simulink model "simFWD_1dof"  (R2021b)
settings: Solver=FixedStepAuto  StartTime=0.0  StopTime=simTime  FixedStep=samplingPeriod/500
values from neighbouring files (symbols this model uses):
  drv = driveNo3    [id_1dof_dyn.m]    (also in id_1dof_static.m)
  dwellTimeInit = 0    [id_1dof_dyn.m]
  frictionInit = Transmission.getFrictionCoeff(velocityInit, kinFriction, strbInf, strbVelocity)    [id_1dof_dyn.m]
  loadInertia = mass*pulleyRad^2    (= 3.84e-05)    [id_1dof_dyn.m]    (also in id_1dof_static.m)
  payload = gravity*mass*pulleyRad    (= 0.01883904)    [id_1dof_dyn.m]    (also in id_1dof_static.m)
  velocityInit = mean(expVelocity(1:5))    [id_1dof_dyn.m]
settings Model: Creator=anestis  LastModifiedBy=Anestis Mablekos
settings SolverCC: AlgebraicLoopSolver=TrustRegion  SolverResetMethod=Robust
settings DataIOCC: ReturnWorkspaceOutputs=off
settings DebuggingCC: SFMachineParentedDataDiag=warning  ArithmeticOperatorsInVariantConditions=warning
settings SFSimCC: SimUseLocalCustomCode=off  CustomCodeUndefinedFunction=UseInterfaceOnly
settings RTWCC: RTWUseLocalCustomCode=off
settings CodeAppCC: StateflowObjectComments=on

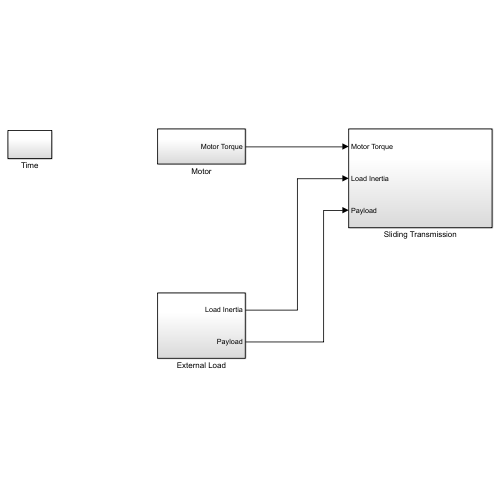
[thumbnail: Simulink's stored preview of the top-level diagram]
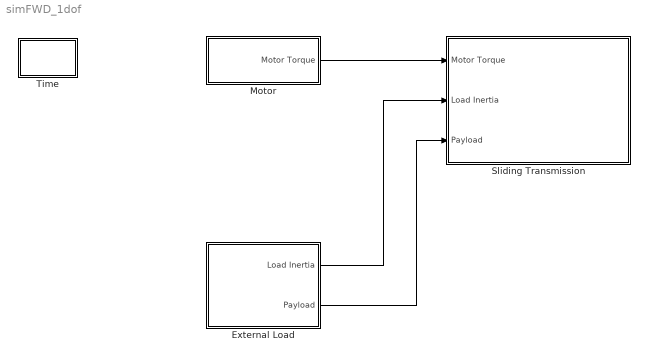
== system simFWD_1dof ==
  External Load : Subsystem
  Motor : Subsystem
  Sliding Transmission : Subsystem
  Time : Subsystem
  wires:
  External Load/1(Load Inertia) -> Sliding Transmission/2(Load Inertia)
  External Load/2(Payload) -> Sliding Transmission/3(Payload)
  Motor/1(Motor Torque) -> Sliding Transmission/1(Motor Torque)

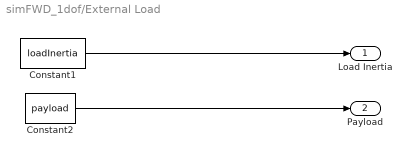
== system simFWD_1dof/External Load ==
  Constant1 : Constant  Value=loadInertia
  Constant2 : Constant  Value=payload
  Load Inertia : Outport
  Payload : Outport  Port=2
  wires:
  Constant1/1 -> Load Inertia/1
  Constant2/1 -> Payload/1

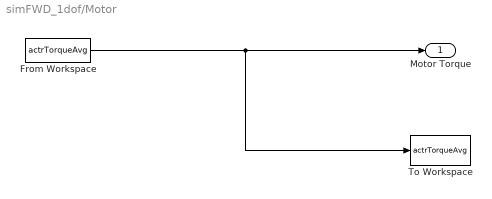
== system simFWD_1dof/Motor ==
  From Workspace : FromWorkspace  VariableName=actrTorqueAvg
  To Workspace : ToWorkspace  VariableName=actrTorqueAvg  SaveFormat=Timeseries  SampleTime=-1
  Motor Torque : Outport
  wires:
  From Workspace/1 -> To Workspace/1, Motor Torque/1

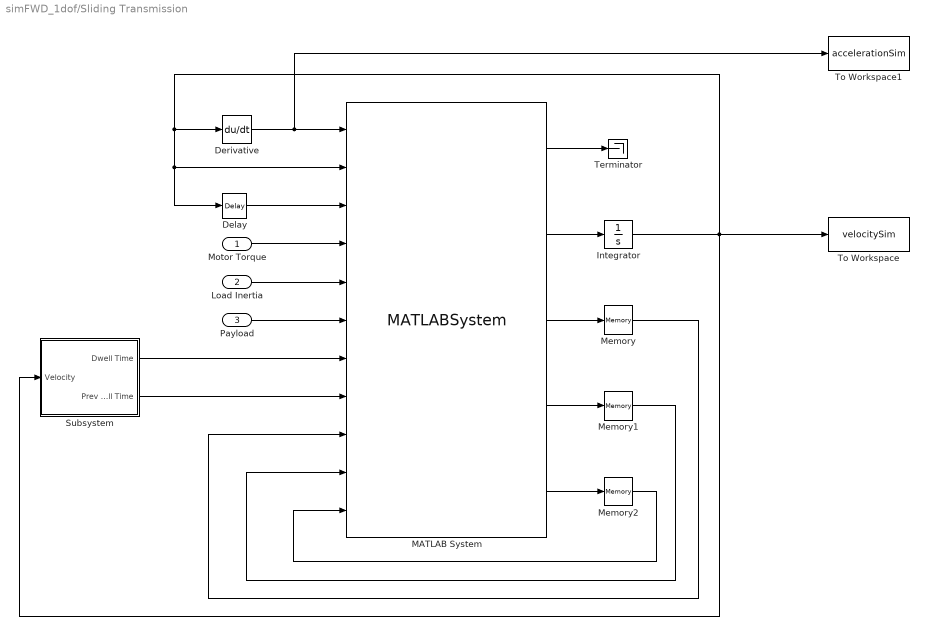
== system simFWD_1dof/Sliding Transmission ==
  Motor Torque : Inport
  Load Inertia : Inport  Port=2
  Payload : Inport  Port=3
  Delay : TransportDelay  DelayTime=drv.friction.memoryCst  InitialOutput=velocityInit
  Derivative : Derivative
  Integrator : Integrator
  MATLAB System : MATLABSystem  System=Transmission  geometry=drv.geometry  preload=drv.preload  friction=drv.friction  inertia=drv.inertia  actuation=drv.actuation  SimulateUsing=Code generation
      mask Type: Transmission
      mask Display:
      | disp('Transmission');
      | port_label('input',1,'acceleration');
      | port_label('input',2,'velocity');
      | port_label('input',3,'velocityD');
      | port_label('input',4,'actrTorque');
      | port_label('input',5,'loadInertia');
      | port_label('input',6,'payload');
      | port_label('input',7,'dwellTime');
      | port_label('input',8,'dwellTimePrev');
      | port_label('input',9,'frictionCoeffPrev');
      | port_label('input',10,'strbFrictionPrev');
      | port_label('input',11,'strbArrivalPrev');
      | port_label('output',1,'torque');
      | port_label('output',2,'acceleration');
      | port_label('output',3,'frictionCoeff');
      | port_label('output',4,'strbFriction');
      | port_label('output',5,'strbArrival');
  Memory : Memory  InitialCondition=frictionInit
  Memory1 : Memory  InitialCondition=drv.friction.strbInf
  Memory2 : Memory  InitialCondition=drv.friction.strbInf
  Subsystem : Subsystem
  Terminator : Terminator
  To Workspace : ToWorkspace  VariableName=velocitySim  SaveFormat=Timeseries  SampleTime=-1
  To Workspace1 : ToWorkspace  VariableName=accelerationSim  SaveFormat=Timeseries  SampleTime=-1
  wires:
  Motor Torque/1 -> MATLAB System/4
  Load Inertia/1 -> MATLAB System/5
  Payload/1 -> MATLAB System/6
  Memory/1 -> MATLAB System/9
  Memory1/1 -> MATLAB System/10
  Delay/1 -> MATLAB System/3
  Memory2/1 -> MATLAB System/11
  Integrator/1 -> Subsystem/1(Velocity), To Workspace/1, Delay/1, MATLAB System/2, Derivative/1
  Derivative/1 -> To Workspace1/1, MATLAB System/1
  MATLAB System/5 -> Memory2/1
  MATLAB System/3 -> Memory/1
  MATLAB System/2 -> Integrator/1
  MATLAB System/1 -> Terminator/1
  MATLAB System/4 -> Memory1/1
  Subsystem/1(Dwell Time) -> MATLAB System/7
  Subsystem/2(Prev Dwell Time) -> MATLAB System/8

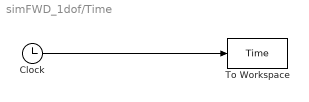
== system simFWD_1dof/Time ==
  Clock : Clock
  To Workspace : ToWorkspace  VariableName=Time  SaveFormat=Timeseries  SampleTime=-1
  wires:
  Clock/1 -> To Workspace/1

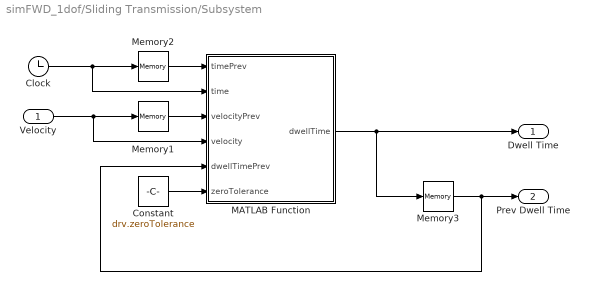
== system simFWD_1dof/Sliding Transmission/Subsystem ==
  Velocity : Inport
  Clock : Clock
  Constant : Constant  Value=drv.zeroTolerance
  MATLAB Function : MATLAB Function  TreatAsAtomicUnit=on
  Memory1 : Memory  InitialCondition=velocityInit
  Memory2 : Memory
  Memory3 : Memory  InitialCondition=dwellTimeInit
  Dwell Time : Outport
  Prev Dwell Time : Outport  Port=2
  wires:
  Memory1/1 -> MATLAB Function/3(velocityPrev)
  Constant/1 -> MATLAB Function/6(zeroTolerance)
  Velocity/1 -> MATLAB Function/4(velocity), Memory1/1
  Memory2/1 -> MATLAB Function/1(timePrev)
  Memory3/1 -> MATLAB Function/5(dwellTimePrev), Prev Dwell Time/1
  Clock/1 -> MATLAB Function/2(time), Memory2/1
  MATLAB Function/1(dwellTime) -> Dwell Time/1, Memory3/1

== matlab function simFWD_1dof/Sliding Transmission/Subsystem/MATLAB Function ==
  data: timePrev input; time input; velocityPrev input; velocity input; dwellTime output; dwellTimePrev input; zeroTolerance input
function dwellTime = fcn(timePrev, time, velocityPrev, velocity, dwellTimePrev, zeroTolerance)

int = time-timePrev;

if abs(velocity) < zeroTolerance
    if abs(velocity-velocityPrev) < zeroTolerance
        dwellTime = int + dwellTimePrev;
    else
        dwellTime = 0;
    end
else
    dwellTime = 0;
end
